simulink model "VehicleSimulation"  (R2018b)
settings: Solver=FixedStepAuto  StartTime=0.0  StopTime=Tsim  FixedStep=Ts  RelTol=1e-6
values from neighbouring files (symbols this model uses):
  Ts = 0.01    [modelFitEDMD.m]
  x0 = xLowLim + rand(nx,Ntraj).*(xUppLim - xLowLim)    [errorAnalysis.m]    (also in simulationEDMD.m = [37.7777; -8.2569; -1.5693])
settings Model: Creator=Marko  LastModifiedBy=Marko

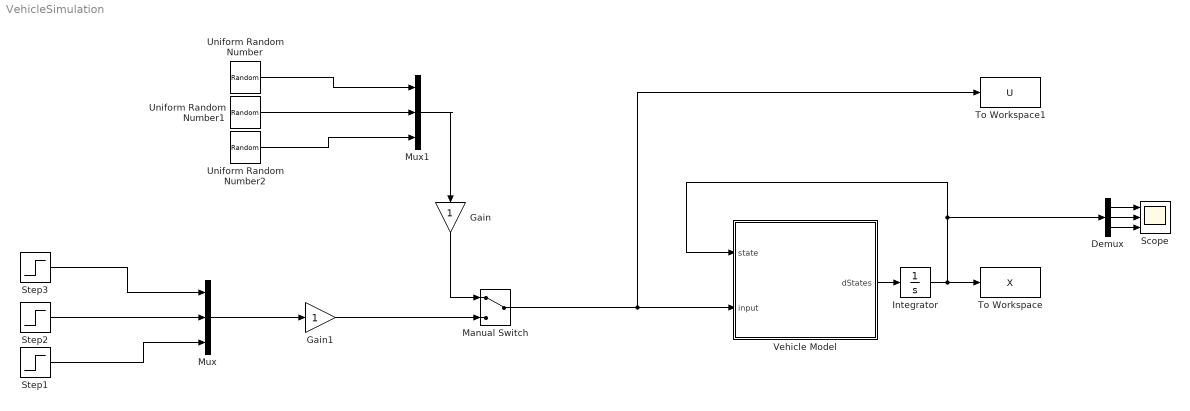
== system VehicleSimulation ==
  Demux : Demux  Outputs=3
  Gain : Gain
  Gain1 : Gain
  Integrator : Integrator  InitialCondition=x0
  Manual Switch : ManualSwitch
  Mux : Mux  Inputs=3
  Mux1 : Mux  Inputs=3
  Scope : Scope  NumInputPorts=3
  Step1 : Step  Time=10  After=50000  SampleTime=0
  Step2 : Step  Time=0.2  After=12000  SampleTime=0
  Step3 : Step  Time=0  After=10000  SampleTime=0
  To Workspace : ToWorkspace  VariableName=X  SampleTime=Ts
  To Workspace1 : ToWorkspace  VariableName=U  SampleTime=Ts
  Uniform Random Number : UniformRandomNumber  Minimum=-50000  Maximum=50000  Seed=12  SampleTime=Ts
  Uniform Random Number1 : UniformRandomNumber  Minimum=-50000  Maximum=50000  Seed=10  SampleTime=Ts
  Uniform Random Number2 : UniformRandomNumber  Minimum=-50000  Maximum=50000  SampleTime=Ts
  Vehicle Model : MATLAB Function  TreatAsAtomicUnit=on
  wires:
  Vehicle Model/1(dStates) -> Integrator/1
  Integrator/1 -> To Workspace/1, Demux/1, Vehicle Model/1(state)
  Step2/1 -> Mux/2
  Step1/1 -> Mux/3
  Uniform Random Number2/1 -> Mux1/3
  Uniform Random Number1/1 -> Mux1/2
  Mux1/1 -> Gain/1
  Manual Switch/1 -> To Workspace1/1, Vehicle Model/2(input)
  Mux/1 -> Gain1/1
  Uniform Random Number/1 -> Mux1/1
  Gain/1 -> Manual Switch/1
  Demux/1 -> Scope/1
  Demux/2 -> Scope/2
  Demux/3 -> Scope/3
  Gain1/1 -> Manual Switch/2
  Step3/1 -> Mux/1

== matlab function VehicleSimulation/Vehicle Model ==
  data: state input; dStates output; input input
function dStates  = BicycleModel(state,input)

% Extract states
vx = state(1);
vy = state(2);
yawRate = state(3);

% Extract inputs
Fxf = input(1);
Fyf = input(2);
Fxr = input(3);

% Load parameters
vehicle = LoadVehicleParameters();

% Vehicle parameters
a = vehicle.a;
b = vehicle.b;
m = vehicle.Mass;
I = vehicle.Izz;

% Air drag parameters
cw = vehicle.cw;
rho = vehicle.rho;
Aw = vehicle.Aw;

% Tyre parameters
Cxf = vehicle.Cxf;
Cyf = vehicle.Cyf;
Cxr = vehicle.Cxr;
Cyr = vehicle.Cyr;

% Lateral velocities
vyf = vy + a*yawRate;
vyr = vy - b*yawRate;
% Longitudinal velocities
vxf = vx;
vxr = vx;

% TYRE VELOCITIES
% Cornering velocities
%vcf = vyf*cos(deltaF) - vxf*sin(deltaF);
vcr = vyr;
% Longitudinal velocities
%vlf = vyf*sin(deltaF) + vxf*cos(deltaF);
vlr = vxr;

% TYRE SLIP ANGLES
%alpha_f = atan2(vcf,vlf);
alpha_r = atan2(vcr,vlr);

% Longitudinal and cornering forces
%Flf = Cxf*sF;
%Flr = Cxr*sR;
%Fcf = -Cyf*alpha_f;
Fcr = -Cyr*alpha_r;

% AXLE FORCES
% Lateral forces
%Fyf = Flf*sin(deltaF) + Fcf*cos(deltaF);
Fyr = Fcr;
% Longitudinal forces
%Fxf = Flf*cos(deltaF) - Fcf*sin(deltaF);
%Fxr = Flr;

dVx = yawRate*vy + 1/m*(-0.5*cw*rho*Aw*sqrt(vx^2+vy^2)*vx + Fxf + Fxr);
dVy = -yawRate*vx + 1/m*(-0.5*cw*rho*Aw*sqrt(vx^2+vy^2)*vy + Fyf + Fyr);
dYawRate = 1/I * (Fyf*a - Fyr*b);

dStates = [dVx; dVy; dYawRate];

end
